simulink model "spindle_model"  (R2016b)
settings: Solver=FixedStepAuto  StartTime=0  StopTime=10  FixedStep=0.001  RelTol=1e-3  EnableMultiTasking=on
settings Model: Creator=Manu  LastModifiedBy=Manu
settings SolverCC: NumberNewtonIterations=2
settings OptimizationCC: LifeSpan=inf
settings DebuggingCC: SFUnexpectedBacktrackingDiag=warning  SFNoUnconditionalDefaultTransitionDiag=warning  SFUnconditionalPathOutOfParentDiag=warning  SFExecutionAtInitializationDiag=none  SFUnreachableStateOrJunctionDiag=warning  SFDanglingTransitionDiag=warning
settings CodeAppCC: CustomSymbolStrSimulinkFcn=$N
settings GRTTargetCC: TargetLangStandard=C89/C90 (ANSI)  GeneratePreprocessorConditionals=Disable all
settings ConfigComp: CovMetricSettings=dw  CovHtmlReporting=on  CovSaveCumulativeToWorkspaceVar=on  CovSaveSingleToWorkspaceVar=on  CovExternalEMLEnable=off

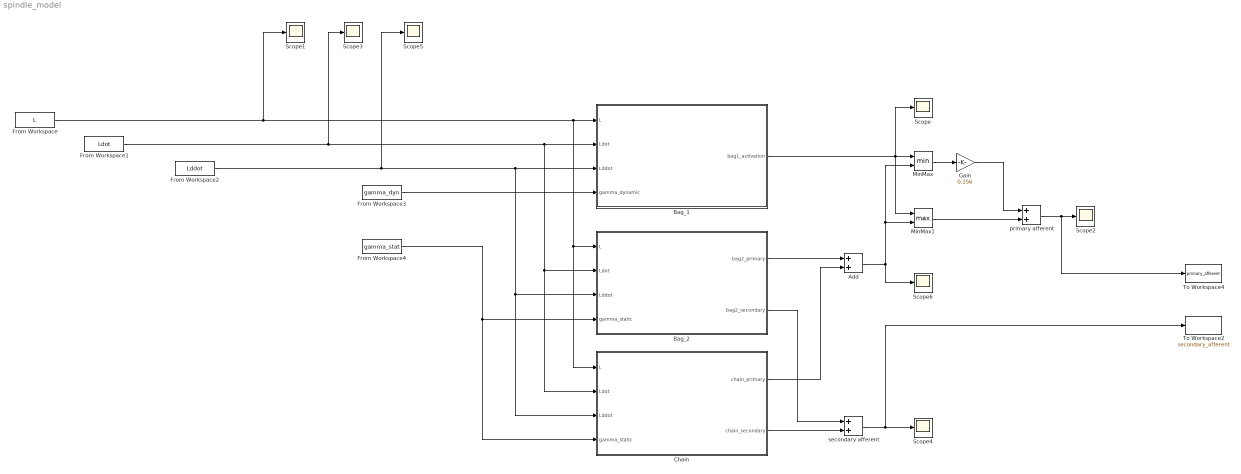
== system spindle_model ==
  Add : Sum
  Bag_1 : Subsystem
  Bag_2 : Subsystem
  Chain : Subsystem
  From Workspace : FromWorkspace  VariableName=L  SampleTime=0
  From Workspace1 : FromWorkspace  VariableName=Ldot  SampleTime=0
  From Workspace2 : FromWorkspace  VariableName=Lddot  SampleTime=0
  From Workspace3 : FromWorkspace  VariableName=gamma_dyn  SampleTime=0
  From Workspace4 : FromWorkspace  VariableName=gamma_stat  SampleTime=0
  Gain : Gain  Gain=0.156
  MinMax : MinMax  Inputs=2
  MinMax1 : MinMax  Function=max  Inputs=2
  Scope{,1..6} (7 alike) : Scope
  To Workspace2 : ToWorkspace  VariableName=secondary_afferent  SaveFormat=Timeseries  SampleTime=-1
  To Workspace4 : ToWorkspace  VariableName=primary_afferent  SaveFormat=Timeseries  SampleTime=-1
  primary afferent : Sum
  secondary afferent : Sum
  wires:
  From Workspace4/1 -> Chain/4(gamma_static), Bag_2/4(gamma_static)
  Bag_2/1(bag2_primary) -> Add/1
  Chain/1(chain_primary) -> Add/2
  Chain/2(chain_secondary) -> secondary afferent/2
  Bag_1/1(bag1_activation) -> Scope/1, MinMax1/1, MinMax/1
  Add/1 -> Scope6/1, MinMax/2, MinMax1/2
  MinMax/1 -> Gain/1
  Gain/1 -> primary afferent/1
  MinMax1/1 -> primary afferent/2
  primary afferent/1 -> To Workspace4/1, Scope2/1
  secondary afferent/1 -> To Workspace2/1, Scope4/1
  From Workspace3/1 -> Bag_1/4(gamma_dynamic)
  From Workspace2/1 -> Scope5/1, Chain/3(Lddot), Bag_2/3(Lddot), Bag_1/3(Lddot)
  From Workspace1/1 -> Chain/2(Ldot), Bag_2/2(Ldot), Bag_1/2(Ldot), Scope3/1
  From Workspace/1 -> Scope1/1, Chain/1(L), Bag_2/1(L), Bag_1/1(L)
  Bag_2/2(bag2_secondary) -> secondary afferent/1

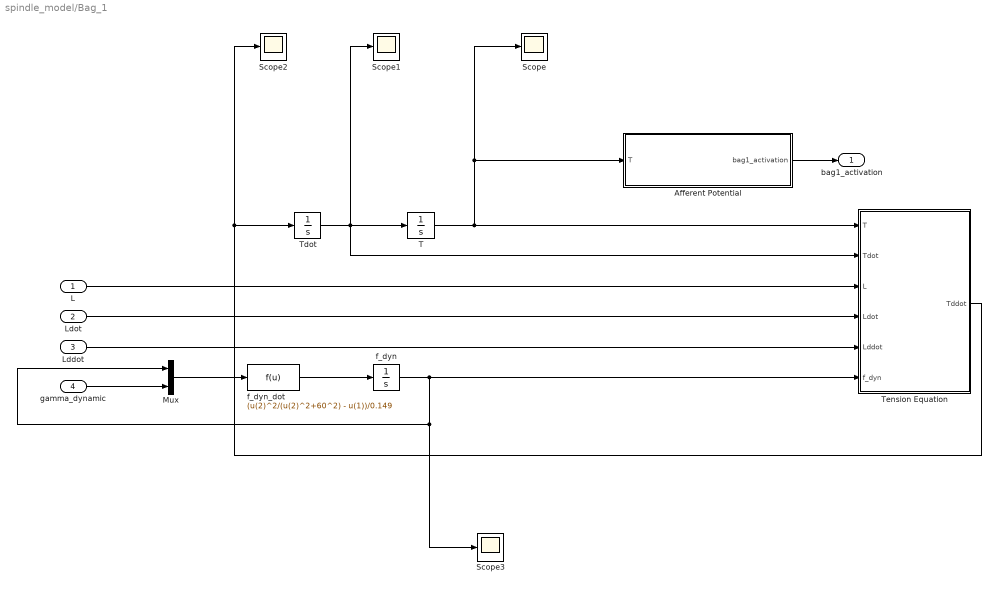
== system spindle_model/Bag_1 ==
  L : Inport
  Ldot : Inport  Port=2
  Lddot : Inport  Port=3
  gamma_dynamic : Inport  Port=4
  Afferent Potential : MATLAB Function  TreatAsAtomicUnit=on
  Mux : Mux  Inputs=2
  Scope{,1..3} (4 alike) : Scope
  T : Integrator
  Tdot : Integrator
  Tension Equation : MATLAB Function  TreatAsAtomicUnit=on
  f_dyn : Integrator
  f_dyn_dot : Fcn  Expr=(u(2)^2/(u(2)^2+60^2) - u(1))/0.149
  bag1_activation : Outport
  wires:
  gamma_dynamic/1 -> Mux/2
  Mux/1 -> f_dyn_dot/1
  f_dyn_dot/1 -> f_dyn/1
  Tdot/1 -> Scope1/1, Tension Equation/2(Tdot), T/1
  T/1 -> Scope/1, Afferent Potential/1(T), Tension Equation/1(T)
  L/1 -> Tension Equation/3(L)
  Ldot/1 -> Tension Equation/4(Ldot)
  Lddot/1 -> Tension Equation/5(Lddot)
  f_dyn/1 -> Scope3/1, Mux/1, Tension Equation/6(f_dyn)
  Tension Equation/1(Tddot) -> Scope2/1, Tdot/1
  Afferent Potential/1(bag1_activation) -> bag1_activation/1

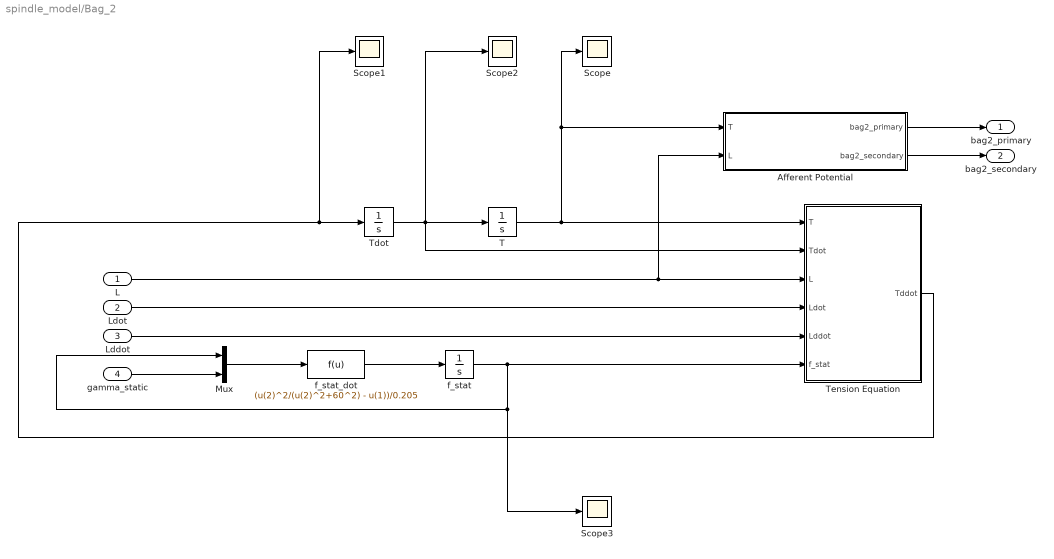
== system spindle_model/Bag_2 ==
  L : Inport
  Ldot : Inport  Port=2
  Lddot : Inport  Port=3
  gamma_static : Inport  Port=4
  Afferent Potential : MATLAB Function  TreatAsAtomicUnit=on
  Mux : Mux  Inputs=2
  Scope{,1..3} (4 alike) : Scope
  T : Integrator
  Tdot : Integrator
  Tension Equation : MATLAB Function  TreatAsAtomicUnit=on
  f_stat : Integrator
  f_stat_dot : Fcn  Expr=(u(2)^2/(u(2)^2+60^2) - u(1))/0.205
  bag2_primary : Outport
  bag2_secondary : Outport  Port=2
  wires:
  gamma_static/1 -> Mux/2
  Mux/1 -> f_stat_dot/1
  f_stat_dot/1 -> f_stat/1
  f_stat/1 -> Mux/1, Scope3/1, Tension Equation/6(f_stat)
  Tdot/1 -> Scope2/1, Tension Equation/2(Tdot), T/1
  T/1 -> Afferent Potential/1(T), Scope/1, Tension Equation/1(T)
  L/1 -> Afferent Potential/2(L), Tension Equation/3(L)
  Ldot/1 -> Tension Equation/4(Ldot)
  Lddot/1 -> Tension Equation/5(Lddot)
  Tension Equation/1(Tddot) -> Scope1/1, Tdot/1
  Afferent Potential/1(bag2_primary) -> bag2_primary/1
  Afferent Potential/2(bag2_secondary) -> bag2_secondary/1

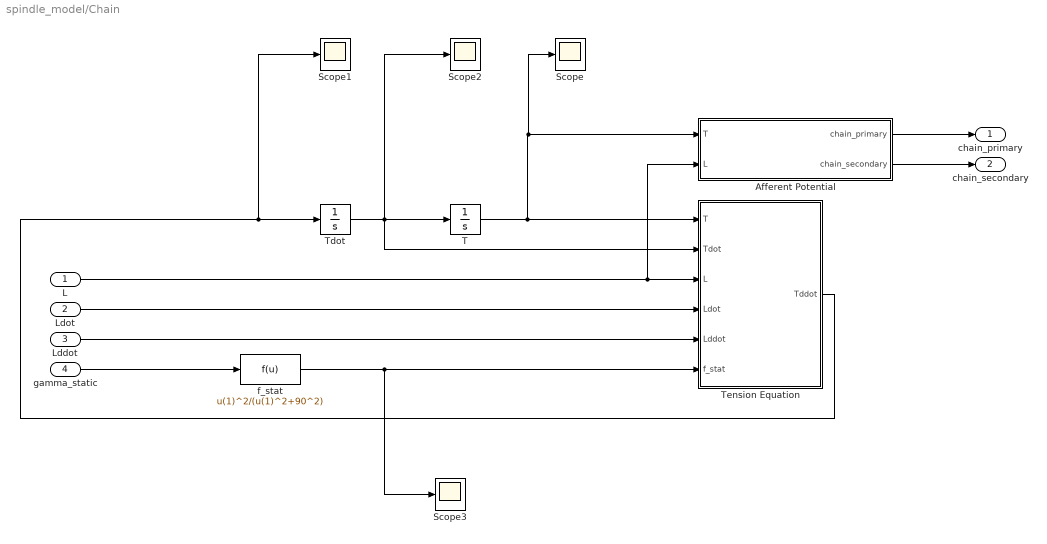
== system spindle_model/Chain ==
  L : Inport
  Ldot : Inport  Port=2
  Lddot : Inport  Port=3
  gamma_static : Inport  Port=4
  Afferent Potential : MATLAB Function  TreatAsAtomicUnit=on
  Scope{,1..3} (4 alike) : Scope
  T : Integrator
  Tdot : Integrator
  Tension Equation : MATLAB Function  TreatAsAtomicUnit=on
  f_stat : Fcn  Expr=u(1)^2/(u(1)^2+90^2)
  chain_primary : Outport
  chain_secondary : Outport  Port=2
  wires:
  f_stat/1 -> Scope3/1, Tension Equation/6(f_stat)
  Tdot/1 -> Scope2/1, Tension Equation/2(Tdot), T/1
  T/1 -> Tension Equation/1(T), Scope/1, Afferent Potential/1(T)
  L/1 -> Afferent Potential/2(L), Tension Equation/3(L)
  Ldot/1 -> Tension Equation/4(Ldot)
  Lddot/1 -> Tension Equation/5(Lddot)
  Tension Equation/1(Tddot) -> Scope1/1, Tdot/1
  Afferent Potential/1(chain_primary) -> chain_primary/1
  Afferent Potential/2(chain_secondary) -> chain_secondary/1
  gamma_static/1 -> f_stat/1

== matlab function spindle_model/Bag_1/Afferent Potential ==
  data: T input; bag1_activation output
function bag1_activation = activation(T)

Ksr = 10.4649;
L0_sr = 0.04;
G = 20000;
LN_sr = 0.0423;

bag1_activation = G*(T/Ksr + L0_sr - LN_sr);

== matlab function spindle_model/Bag_1/Tension Equation ==
  data: T input; Tddot output; Tdot input; L input; Ldot input; Lddot input; f_dyn input
function Tddot = Tddot(T,Tdot,L,Ldot,Lddot,f_dyn)

Ksr = 10.4649;
Kpr = 0.15;
M = 0.0002;
CL = 1;
CS = 0.42;
a = 0.3;
R = 0.46;
L0_sr = 0.04;
L0_pr = 0.76;

beta = 0.0605 + 0.2592*f_dyn;
gamma = 0.0289*f_dyn;

if Ldot-Tdot/Ksr>0
	C = CL;
else
	C = CS;
end

Tddot = M*Lddot + gamma - T;
Tddot = Tddot + Kpr*(L - L0_sr - T/Ksr - L0_pr);
Tddot = Tddot + C*beta*sign(Ldot - Tdot/Ksr)*abs(Ldot - Tdot/Ksr)^a*(L-L0_sr-T/Ksr-R);
Tddot = Tddot*Ksr/M;

== matlab function spindle_model/Bag_2/Afferent Potential ==
  data: T input; bag2_primary output; bag2_secondary output; L input
function [bag2_primary,bag2_secondary] = activation(T,L)

Ksr = 10.4649;
L0_sr = 0.04;
L0_pr = 0.76;
G1 = 10000;
G2 = 7250;
LN_sr = 0.0423;
LN_pr = 0.89;
X = 0.7;
Lsec = 0.04;

bag2_primary = G1*(T/Ksr + L0_sr - LN_sr);
bag2_secondary = G2*(X*Lsec/L0_sr*(T/Ksr + L0_sr - LN_sr) + (1-X)*Lsec/L0_pr*(L - T/Ksr - L0_sr - LN_pr));

== matlab function spindle_model/Bag_2/Tension Equation ==
  data: T input; Tddot output; Tdot input; L input; Ldot input; Lddot input; f_stat input
function Tddot = Tddot(T,Tdot,L,Ldot,Lddot,f_stat)

Ksr = 10.4649;
Kpr = 0.15;
M = 0.0002;
CL = 1;
CS = 0.42;
a = 0.3;
R = 0.46;
L0_sr = 0.04;
L0_pr = 0.76;

beta = 0.0822 - 0.0460*f_stat;
gamma = 0.0636*f_stat;

if Ldot-Tdot/Ksr>0
	C = CL;
else
	C = CS;
end

Tddot = M*Lddot + gamma - T;
Tddot = Tddot + Kpr*(L - L0_sr - T/Ksr - L0_pr);
Tddot = Tddot + C*beta*sign(Ldot - Tdot/Ksr)*abs(Ldot - Tdot/Ksr)^a*(L-L0_sr-T/Ksr-R);
Tddot = Tddot*Ksr/M;

== matlab function spindle_model/Chain/Afferent Potential ==
  data: T input; chain_primary output; chain_secondary output; L input
function [chain_primary,chain_secondary] = activation(T,L)

Ksr = 10.4649;
L0_sr = 0.04;
L0_pr = 0.76;
G1 = 10000;
G2 = 7250;
LN_sr = 0.0423;
LN_pr = 0.89;
X = 0.7;
Lsec = 0.04;

chain_primary = G1*(T/Ksr + L0_sr - LN_sr);
chain_secondary = G2*(X*Lsec/L0_sr*(T/Ksr + L0_sr - LN_sr) + (1-X)*Lsec/L0_pr*(L - T/Ksr - L0_sr - LN_pr));

== matlab function spindle_model/Chain/Tension Equation ==
  data: T input; Tddot output; Tdot input; L input; Ldot input; Lddot input; f_stat input
function Tddot = Tddot(T,Tdot,L,Ldot,Lddot,f_stat)

Ksr = 10.4649;
Kpr = 0.15;
M = 0.0002;
CL = 1;
CS = 0.42;
a = 0.3;
R = 0.46;
L0_sr = 0.04;
L0_pr = 0.76;

beta = 0.0822 - 0.0690*f_stat;
gamma = 0.0954*f_stat;

if Ldot-Tdot/Ksr>0
	C = CL;
else
	C = CS;
end

Tddot = M*Lddot + gamma - T;
Tddot = Tddot + Kpr*(L - L0_sr - T/Ksr - L0_pr);
Tddot = Tddot + C*beta*sign(Ldot - Tdot/Ksr)*abs(Ldot - Tdot/Ksr)^a*(L-L0_sr-T/Ksr-R);
Tddot = Tddot*Ksr/M;
